simulink model "Closest_point_calculate"  (R2021a)
settings: configuration reference "AION_IDS_Speedgoat" (kept outside this file)
libraries: simulink x1
settings Model: DataDictionary=Closest_Point_Calculate.sldd  Creator=xinrui  LastModifiedBy=Administrator
settings ConfigSetRef: SourceName=AION_IDS_Speedgoat

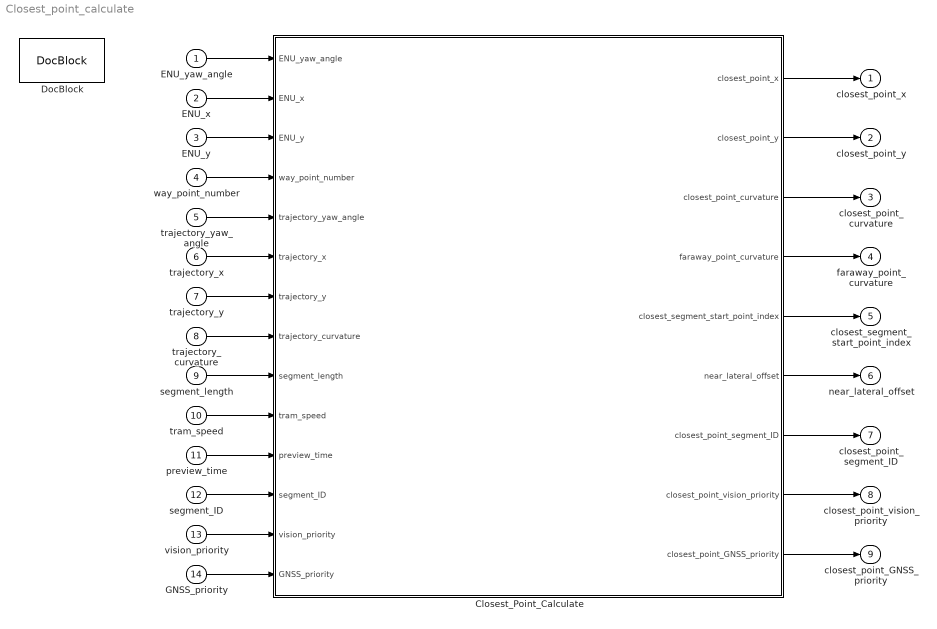
== system Closest_point_calculate ==
  ENU_yaw_angle : Inport  OutDataTypeStr=double  PortDimensions=1
  ENU_x : Inport  Port=2  OutDataTypeStr=double  PortDimensions=1
  ENU_y : Inport  Port=3  OutDataTypeStr=double  PortDimensions=1
  way_point_number : Inport  Port=4  OutDataTypeStr=double  PortDimensions=1
  trajectory_yaw_angle : Inport  Port=5  OutDataTypeStr=double
  trajectory_x : Inport  Port=6  OutDataTypeStr=double
  trajectory_y : Inport  Port=7  OutDataTypeStr=double
  trajectory_curvature : Inport  Port=8  OutDataTypeStr=double
  segment_length : Inport  Port=9  OutDataTypeStr=double
  tram_speed : Inport  Port=10  OutDataTypeStr=double  PortDimensions=1
  preview_time : Inport  Port=11  OutDataTypeStr=double  PortDimensions=1
  segment_ID : Inport  Port=12  OutDataTypeStr=double
  vision_priority : Inport  Port=13  OutDataTypeStr=double
  GNSS_priority : Inport  Port=14  OutDataTypeStr=double
  Closest_Point_Calculate : MATLAB Function  TreatAsAtomicUnit=on
  DocBlock : simulink/Model-Wide Utilities/DocBlock  DocumentType=HTML  mask(DocBlock){}
      mask Display:
      | plot([.8 0 0 1 1 .8 .8 1],[1 1 0 0 .8 1 .8 .8]);
      | text(.5,.6,'CHANGELOG','horizontalalignment','center');
      | text(.95,.05,get_param(gcb,'DocumentType'),'verticalalignment','bottom','horizontalalignment','right');
  closest_point_x : Outport  OutDataTypeStr=double  PortDimensions=1
  closest_point_y : Outport  Port=2  OutDataTypeStr=double  PortDimensions=1
  closest_point_curvature : Outport  Port=3  OutDataTypeStr=double  PortDimensions=1
  faraway_point_curvature : Outport  Port=4  OutDataTypeStr=double  PortDimensions=1
  closest_segment_start_point_index : Outport  Port=5  OutDataTypeStr=double  PortDimensions=1
  near_lateral_offset : Outport  Port=6  OutDataTypeStr=double  PortDimensions=1
  closest_point_segment_ID : Outport  Port=7  OutDataTypeStr=double  PortDimensions=1
  closest_point_vision_priority : Outport  Port=8  OutDataTypeStr=double  PortDimensions=1
  closest_point_GNSS_priority : Outport  Port=9  OutDataTypeStr=double  PortDimensions=1
  wires:
  ENU_yaw_angle/1 -> Closest_Point_Calculate/1(ENU_yaw_angle)
  ENU_x/1 -> Closest_Point_Calculate/2(ENU_x)
  ENU_y/1 -> Closest_Point_Calculate/3(ENU_y)
  way_point_number/1 -> Closest_Point_Calculate/4(way_point_number)
  trajectory_yaw_angle/1 -> Closest_Point_Calculate/5(trajectory_yaw_angle)
  trajectory_x/1 -> Closest_Point_Calculate/6(trajectory_x)
  trajectory_y/1 -> Closest_Point_Calculate/7(trajectory_y)
  trajectory_curvature/1 -> Closest_Point_Calculate/8(trajectory_curvature)
  segment_length/1 -> Closest_Point_Calculate/9(segment_length)
  tram_speed/1 -> Closest_Point_Calculate/10(tram_speed)
  preview_time/1 -> Closest_Point_Calculate/11(preview_time)
  Closest_Point_Calculate/1(closest_point_x) -> closest_point_x/1
  Closest_Point_Calculate/2(closest_point_y) -> closest_point_y/1
  Closest_Point_Calculate/3(closest_point_curvature) -> closest_point_curvature/1
  Closest_Point_Calculate/4(faraway_point_curvature) -> faraway_point_curvature/1
  Closest_Point_Calculate/5(closest_segment_start_point_index) -> closest_segment_start_point_index/1
  Closest_Point_Calculate/6(near_lateral_offset) -> near_lateral_offset/1
  Closest_Point_Calculate/7(closest_point_segment_ID) -> closest_point_segment_ID/1
  Closest_Point_Calculate/8(closest_point_vision_priority) -> closest_point_vision_priority/1
  Closest_Point_Calculate/9(closest_point_GNSS_priority) -> closest_point_GNSS_priority/1
  segment_ID/1 -> Closest_Point_Calculate/12(segment_ID)
  vision_priority/1 -> Closest_Point_Calculate/13(vision_priority)
  GNSS_priority/1 -> Closest_Point_Calculate/14(GNSS_priority)

== matlab function Closest_point_calculate/Closest_Point_Calculate ==
  data: ENU_yaw_angle input double size=1; closest_point_x output double size=1; ENU_x input double size=1; ENU_y input double size=1; way_point_number input double size=1; closest_point_y output double size=1; closest_point_curvature output double size=1; faraway_point_curvature output double size=1; closest_segment_start_point_index output double size=1; near_lateral_offset output double size=1; trajectory_yaw_angle input double size=MAX_TRAJECTORY_WAY_POINT_NUMBER; trajectory_x input double size=MAX_TRAJECTORY_WAY_POINT_NUMBER; trajectory_y input double size=MAX_TRAJECTORY_WAY_POINT_NUMBER; trajectory_curvature input double size=MAX_TRAJECTORY_WAY_POINT_NUMBER; segment_length input double size=MAX_TRAJECTORY_WAY_POINT_NUMBER; tram_speed input double size=1; preview_time input double size=1; segment_ID input double size=MAX_TRAJECTORY_WAY_POINT_NUMBER; vision_priority input double size=MAX_TRAJECTORY_WAY_POINT_NUMBER; GNSS_priority input double size=MAX_TRAJECTORY_WAY_POINT_NUMBER; closest_point_segment_ID output double size=1; closest_point_vision_priority output double size=1; closest_point_GNSS_priority output double size=1
% 求参考轨迹上的最近点
function [closest_point_x, closest_point_y, closest_point_curvature, ...
    faraway_point_curvature, closest_segment_start_point_index, ...
    near_lateral_offset, closest_point_segment_ID, closest_point_vision_priority, ...
    closest_point_GNSS_priority] = Closest_point_calculate(ENU_yaw_angle, ENU_x, ...
    ENU_y, way_point_number, trajectory_yaw_angle, trajectory_x, ...
    trajectory_y, trajectory_curvature, segment_length, tram_speed, preview_time, ...
    segment_ID, vision_priority, GNSS_priority)
%   1.输入参数：
%       (1)ENU_yaw_angle                        东北天坐标系下当前点横摆角，deg
%       (2)ENU_x                                东北天坐标系下当前点x坐标，m
%       (3)ENU_y                                东北天坐标系下当前点y坐标，m
%       (4)way_point_number                     局部路径路点个数
%       (5)trajectory_yaw_angle                 局部路径横摆角数组，deg，有效数据数量为way_point_number
%       (6)trajectory_x                         局部路径x坐标数组，m，有效数据数量为way_point_number
%       (7)trajectory_y                         局部路径y坐标数组，m，有效数据数量为way_point_number
%       (8)trajectory_curvature                 局部路径曲率数组，1/m，有效数据数量为way_point_number
%       (9)segment_length                       路点间隔数组，m，有效数据数量为way_point_number
%       (10)tram_speed                          整车车速，m/s
%       (11)preview_time                        预瞄时间，s
%       (12)segment_ID                          区间代号数组，无量纲，有效数据数量为way_point_number
%       (13)vision_priority                     视觉循迹优先级数组，无量纲，有效数据数量为way_point_number
%       (14)GNSS_priority                       GNSS循迹优先级数组，无量纲，有效数据数量为way_point_number
%   2.输出参数：
%       (1)closest_point_x                      最近点x坐标，m
%       (2)closest_point_y                      最近点y坐标，m
%       (3)closest_point_curvature              最近点曲率，1/m
%       (4)faraway_point_curvature              远处路点曲率，1/m
%       (5)closest_segment_start_point_index    最近路点线段起始点索引
%       (6)near_lateral_offset                  近处横向偏差，m
%       (7)closest_point_segment_ID             最近点区间代号，无量纲
%       (8)closest_point_vision_priority        最近点视觉循迹优先级，无量纲
%       (9)closest_point_GNSS_priority          最近点GNSS循迹优先级，无量纲

%% 静态变量声明及初始化
% 上周期最近点x坐标
persistent closest_point_x_previous;
if isempty(closest_point_x_previous)
   closest_point_x_previous = 0;
end

% 上周期最近点y坐标
persistent closest_point_y_previous;
if isempty(closest_point_y_previous)
   closest_point_y_previous = 0;
end

% 上周期最近点曲率
persistent closest_point_curvature_previous;
if isempty(closest_point_curvature_previous)
   closest_point_curvature_previous = 0;
end

%% 初始化
closest_point_x = closest_point_x_previous;
closest_point_y = closest_point_y_previous;
closest_point_curvature = closest_point_curvature_previous;
faraway_point_curvature = 0;
closest_segment_start_point_index = 1;
near_lateral_offset = sqrt((ENU_x - closest_point_x_previous) ^ 2 + (...
    ENU_y - closest_point_y_previous) ^ 2);
closest_point_segment_ID = 0;
closest_point_vision_priority = 0;
closest_point_GNSS_priority = 0;

% 构造轨迹结构体
trajectory.ENU_yaw_angle = trajectory_yaw_angle;
trajectory.ENU_x = trajectory_x;
trajectory.ENU_y = trajectory_y;
trajectory.curvature = trajectory_curvature;
trajectory.segment_length = segment_length;

%% 合法性判断
% 路径点数少于3个时无法使用向量投影法搜索最近点，直接使用上周期的数值输出
if 3 > way_point_number
    return;
end

%% 搜索最近点信息
% 将上周期最近路点线段起始点索引强制设为1，因为最近点正常情况下应该就在第1个点
[closest_point_x, closest_point_y, closest_point_curvature, ...
    closest_segment_start_point_index, near_lateral_offset] = ...
    Trajectory_closest_point_info_get_m(ENU_yaw_angle, ENU_x, ENU_y, trajectory, 1);

%% 输出最近点前方指定路点的曲率
% 计算从最近路点开始向前累计弧长大于等于v*t的路点索引
cumulative_length = 0;
index = closest_segment_start_point_index + 1;
faraway_distance = tram_speed * preview_time;
while way_point_number > index && faraway_distance > cumulative_length
    cumulative_length = cumulative_length + segment_length(index);
    index = index + 1;
end

% 获取满足条件的远处路点曲率
faraway_point_curvature = trajectory_curvature(index);

%% 输出最近点附加属性
closest_point_segment_ID = segment_ID(closest_segment_start_point_index);
closest_point_vision_priority = vision_priority(closest_segment_start_point_index);
closest_point_GNSS_priority = GNSS_priority(closest_segment_start_point_index);

%% 相邻周期数据更新
closest_point_x_previous = closest_point_x;
closest_point_y_previous = closest_point_y;
closest_point_curvature_previous = closest_point_curvature;

end
